simulink model "Verifica_LQR_20022026"  (R2025b)
settings: Solver=VariableStepAuto  StartTime=0.0  StopTime=30.0  RelTol=1e-3
values from neighbouring files (symbols this model uses):
  A = double(subs(A_sym, p_eq_instabile, val_instabili))    [SvolgimentoEsame.m]
  B = double(subs(B_sym, p_eq_instabile, val_instabili))    [SvolgimentoEsame.m]
undefined symbols (not defined in the file or in its folder): C_tot, D_tot, K_LQR_i, K_LQR_x, x_ref_lqr
settings Model: Creator=salvo  LastModifiedBy=salvo

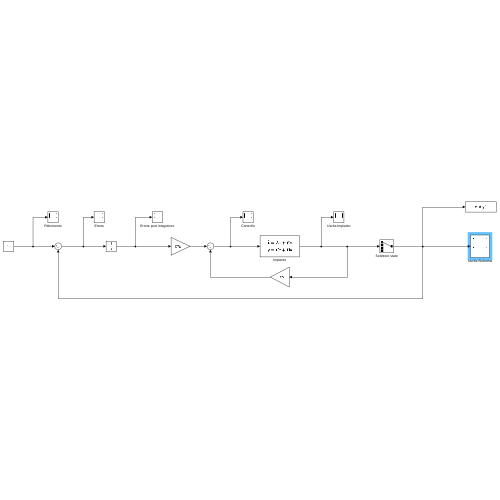
[thumbnail: Simulink's stored preview of the top-level diagram]
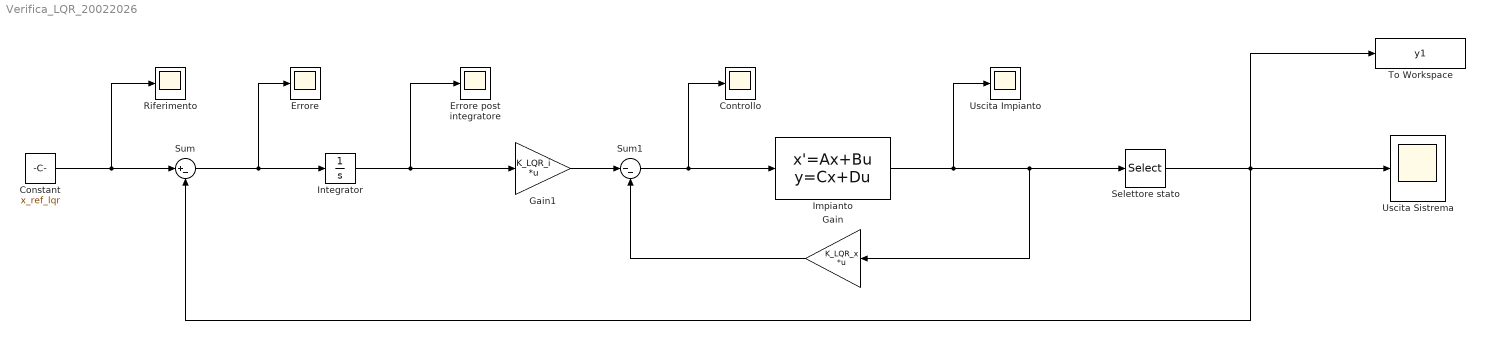
== system Verifica_LQR_20022026 ==
  Constant : Constant  Value=x_ref_lqr
  Controllo : Scope
      settings: DataLoggingVariableName=ScopeData4
  Errore : Scope
      settings: DataLoggingVariableName=ScopeData6
  Errore post integratore : Scope
      settings: DataLoggingVariableName=ScopeData2
  Gain : Gain  Gain=K_LQR_x  Multiplication=Matrix(K*u)
  Gain1 : Gain  Gain=K_LQR_i  Multiplication=Matrix(K*u)
  Impianto : StateSpace  A=A  B=B  C=C_tot  D=D_tot  InitialCondition=0
  Integrator : Integrator
  Riferimento : Scope
  Selettore stato : Selector  InputPortWidth=4  IndexOptions=Index vector (dialog)  Indices=1  OutputSizes=1
  Sum : Sum  Inputs=|+-
  Sum1 : Sum  Inputs=|--
  To Workspace : ToWorkspace  VariableName=y1  SaveFormat=Timeseries  SampleTime=-1
  Uscita Impianto : Scope
      settings: DataLoggingVariableName=ScopeData5
  Uscita Sistrema : Scope
      settings: ActiveDisplayYMinimum=-0.032656465159660718  ActiveDisplayYMaximum=0.28071884423872212
  wires:
  Constant/1 -> Sum/1, Riferimento/1
  Sum/1 -> Integrator/1, Errore/1
  Integrator/1 -> Errore post integratore/1, Gain1/1
  Gain1/1 -> Sum1/1
  Gain/1 -> Sum1/2
  Impianto/1 -> Uscita Impianto/1, Selettore stato/1, Gain/1
  Sum1/1 -> Controllo/1, Impianto/1
  Selettore stato/1 -> To Workspace/1, Sum/2, Uscita Sistrema/1
